simulink model "microcontroller"  (R2024b)
settings: Solver=FixedStepDiscrete  StartTime=0.0  StopTime=inf  RelTol=1e-3  EnableMultiTasking=on
values from neighbouring files (symbols this model uses):
  ac_curr_sens_offset = 1.252    [parameters.m]
  ac_curr_sens_slope = 20.39465588 * 1    (= 20.39465588)    [parameters.m]
  ac_volt_sens_offset = 1.51    [parameters.m]
  ac_volt_sens_slope = 33.33 * 1.00    (= 33.33)    [parameters.m]
  adc_intercept = 0.005546262    [parameters.m]
  adc_slope = 0.000812146    [parameters.m]
  adc_slope_volt = 0.00081 * 1.0    (= 0.00081)    [parameters.m]
  dc_volt_sens_offset = 0.981    [parameters.m]
  dc_volt_sens_slope = 15.122 * 1.0    (= 15.122)    [parameters.m]
  F28M35_freq = 150e6    (= 150000000)    [parameters.m]
  Fs = 20e3    (= 20000)    [parameters.m]
  KI_curr_d = KP_curr_d * Wp1_in    [pi_tuning.m]
  KI_curr_q = KI_curr_d    [pi_tuning.m]
  Ki_pll = 10000    [parameters.m]
  KI_q = C_q_ctrl.Ki    [pi_tuning.m]
  KI_volt = C_volt.Ki    [pi_tuning.m]
  KP_curr_d = Wbi / (DCGain_id * Wp1_in)    [pi_tuning.m]
  KP_curr_q = KP_curr_d    [pi_tuning.m]
  Kp_pll = 500    [parameters.m]
  KP_q = C_q_ctrl.Kp    [pi_tuning.m]
  KP_volt = C_volt.Kp    [pi_tuning.m]
  P = 0.041    [parameters.m]
  rdc = Vdc^2 / P    (= 21951.2195122)    [parameters.m]
  Vdc = 30    [parameters.m]
  wn = 2*pi*60    (= 376.991118431)    [parameters.m]
  Zl = w * Lc    (= 0.957557440814)    [parameters.m]
undefined symbols (not defined in the file or in its folder): Down, GPTRIP1SEL, TZ1, Up
libraries: slpidlib x4, c2802xlib x4, c2000lib x1
settings Model: ExtModeTrigDuration=8  Creator=Asus  LastModifiedBy=Asus
settings SolverCC: AutoInsertRateTranBlk=on
settings OptimizationCC: DefaultParameterBehavior=Inlined  DefaultUnderspecifiedDataType=single  EnhancedBackFolding=on  PassReuseOutputArgsAs=Individual arguments  MaxStackSize=768  OptimizeBlockOrder=speed  DifferentSizesBufferReuse=on  OptimizationCustomize=off  EfficientTunableParamExpr=on
settings DebuggingCC: ParameterTunabilityLossMsg=error
settings HardwareCC: ProdBitPerChar=16  ProdBitPerInt=16  ProdBitPerPointer=32  ProdBitPerSizeT=32  ProdBitPerPtrDiffT=32  ProdLargestAtomicInteger=Integer  ProdLargestAtomicFloat=None  ProdWordSize=16  ProdLongLongMode=on  ProdHWDeviceType=Texas Instruments->C2000
settings SFSimCC: MATLABDynamicMemAlloc=off
settings RTWCC: Description=Embedded Coder  SystemTargetFile=ert.tlc  HardwareBoard=TI Concerto F28M35x (C28x)  TemplateMakefile=ert_default_tmf  GenerateReport=on  Toolchain=Texas Instruments Code Composer Studio (C2000)  LaunchReport=on  CodeProfilingSaveOptions=MetricsOnly
settings RTWCC: CustomInitializer=|
  | InitAdc1();
  | EALLOW;
  | Adc1Regs.ADCCTL2.bit.ADCNONOVERLAP = 1; // Enable non-overlap mode i.e.
  | // conversion and future sampling
  | // events don’t overlap
  | Adc1Regs.ADCCTL1.bit.INTPULSEPOS = 1; // ADCINT1 trips after AdcResults latch
  | Adc1Regs.ADCSOC0CTL.bit.CHSEL = 0; // set SOC0 channel select to ADC1in_A0
  | AnalogSysctrlRegs.TRIG1SEL.all = 1; // Assigning TINT0 to ADC-TRIGGER 1
  | Adc1Regs.ADCSOC0CTL.bit.TRIGSEL = 5; // Set SOC0 start trigger to
  | // ADC Trigger 1 of the ADC
  | Adc1Regs.ADCSOC0CTL.bit.ACQPS = 6; // set SOC0 S/H Window to 7 ADC
  | // Clock Cycles, (6 ACQPS + 1)
  | EDIS;
  | 
  | EALLOW;
  | 
  | // SOC1: ADC1IN_A2
  | Adc1Regs.ADCSOC1CTL.bit.CHSEL = 2;        // Channel A2
  | Adc1Regs.ADCSOC1CTL.bit.TRIGSEL = 5;      // Trigger 1 (TINT0 from ePWM1)
  | Adc1Regs.ADCSOC1CTL.bit.ACQPS = 6;        // Acquisition window
  | 
  | // SOC2: ADC1IN_A3
  | Adc1Regs.ADCSOC2CTL.bit.CHSEL = 3;        // Channel A3
  | Adc1Regs.ADCSOC2CTL.bit.TRIGSEL = 5;      // Trigger 1 (TINT0 from ePWM1)
  | Adc1Regs.ADCSOC2CTL.bit.ACQPS = 6;        // Acquisition window
  | 
  | EDIS;
settings CodeAppCC: ForceParamTrailComments=on  IgnoreCustomStorageClasses=off  OperatorAnnotations=on  SimulinkDataObjDesc=on  SFDataObjDesc=on  InsertBlockDesc=on
settings ERTTargetCC: CodeReplacementLibrary=TI C28x  SupportContinuousTime=on  ExtModeTransport=4  ExtModeStaticAlloc=on  ExtModeAutomaticAllocSize=off  ExtModeStaticAllocSize=2000  ExtModeMexFile=ext_xcp  ExtModeIntrfLevel=Level2 - Open

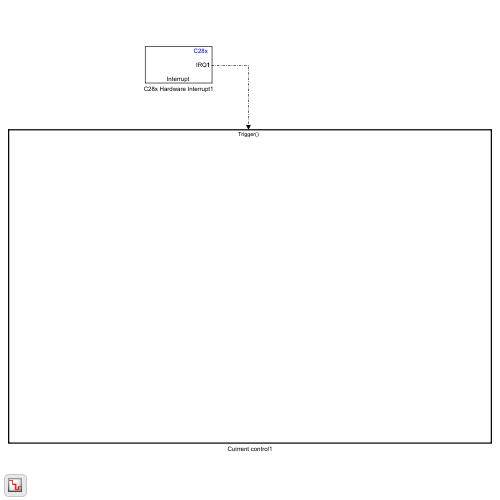
[thumbnail: Simulink's stored preview of the top-level diagram]
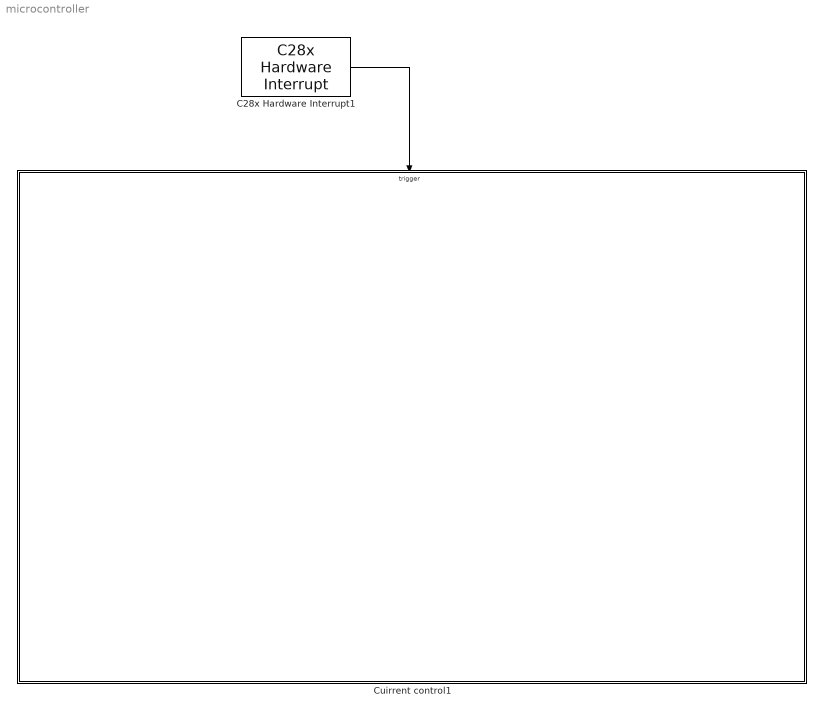
== system microcontroller ==
  C28x Hardware Interrupt1 : c2000lib/Scheduling/C28x Hardware Interrupt  irqnumbers=[1]  pienumbers=[1]  irqpriorities=[30]  irqpreempts=[0]  showinput=off  dspchiptype=C280X
  Cuirrent control1 : Subsystem  TreatAsAtomicUnit=on
  wires:
  C28x Hardware Interrupt1/1 -> Cuirrent control1/Trigger

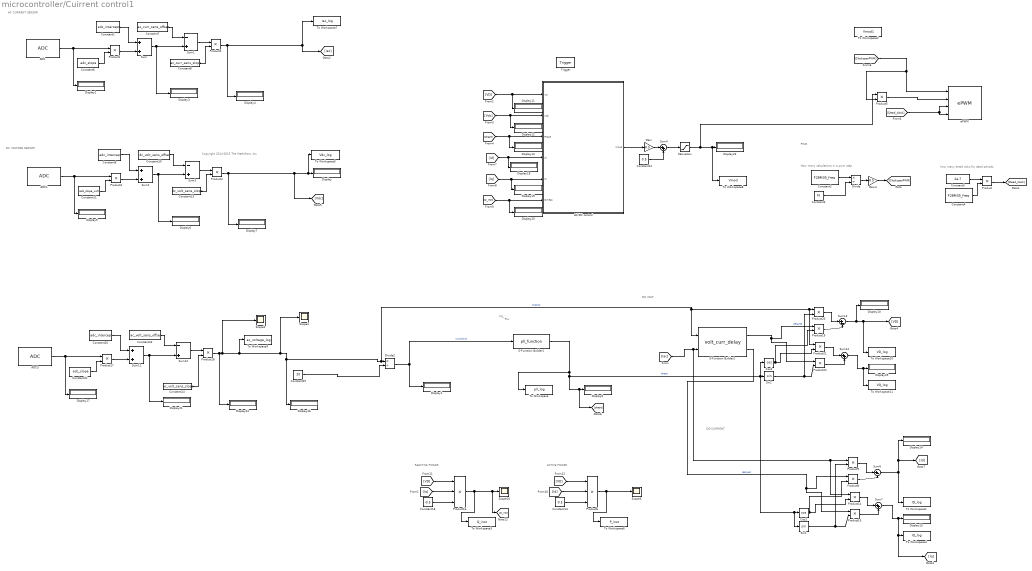
== system microcontroller/Cuirrent control1 ==
  note: PLL
  note: PLL
  note: how many break ticks for dead periods
  note: PWM
  note: How many calculations in a pwm step
  note: AC CURRENT SENSOR
  note: DC VOLTAGE SENSOR
  note: Copyright 2014-2015 The MathWors, Inc.
  note: DQ CURRENT
  note: REACTIVE POWER
  note: DQ VOLT
  note: ACTIVE POWER
  Trigger : TriggerPort  TriggerType=function-call  VariantControl=(inherit)  PortDimensions=1
  AC/DC control : Subsystem
  ADC : c2802xlib/ADC  blkParamProc=Concerto  ADCModule=1  samplingMode=Single sample mode  ADCResolution=12-bit (Single-ended input)  useSOC1=SOC0  useSOC2=SOC0_SOC1  SOCAcquisitionWindow=7  SOCTriggerSource=ePWM1_ADCSOCA  SOCInterruptTrigger=No ADCINT  Ts=-1  dType=uint16  postInterrupt=off  interruptSel=ADCINT1  ADCINTContinuous=off  endma=off  chdma=1  conv1=ADCINA0  conv2=ADCINA0 and ADCINB0  conv1_Type4=ADCIN0  conv2_Type4=ADCIN0 and ADCIN1
      settings: LibrarySourceBlock=f28M35x_C28x_lib/ADC
  ADC1 : c2802xlib/ADC  blkParamProc=Concerto  ADCModule=1  samplingMode=Single sample mode  ADCResolution=12-bit (Single-ended input)  useSOC1=SOC1  useSOC2=SOC0_SOC1  SOCAcquisitionWindow=7  SOCTriggerSource=ePWM1_ADCSOCA  SOCInterruptTrigger=No ADCINT  Ts=-1  dType=uint16  postInterrupt=off  interruptSel=ADCINT1  ADCINTContinuous=off  endma=off  chdma=1  conv1=ADCINA2  conv2=ADCINA0 and ADCINB0  conv1_Type4=ADCIN0  conv2_Type4=ADCIN0 and ADCIN1
      settings: LibrarySourceBlock=f28M35x_C28x_lib/ADC
  ADC3 : c2802xlib/ADC  blkParamProc=Concerto  ADCModule=1  samplingMode=Single sample mode  ADCResolution=12-bit (Single-ended input)  useSOC1=SOC2  useSOC2=SOC0_SOC1  SOCAcquisitionWindow=7  SOCTriggerSource=ePWM1_ADCSOCA  SOCInterruptTrigger=No ADCINT  Ts=-1  dType=uint16  postInterrupt=on  interruptSel=ADCINT1  ADCINTContinuous=off  endma=off  chdma=1  conv1=ADCINA3  conv2=ADCINA0 and ADCINB0  conv1_Type4=ADCIN0  conv2_Type4=ADCIN0 and ADCIN1
      settings: LibrarySourceBlock=f28M35x_C28x_lib/ADC
  Constant1 : Constant  Value=adc_intercept
  Constant10 : Constant  Value=dc_volt_sens_offset
  Constant11 : Constant  Value=adc_slope_volt
  Constant12 : Constant  Value=0.5
  Constant13 : Constant  Value=dc_volt_sens_slope
  Constant14 : Constant  Value=0.5
  Constant18 : Constant  Value=-0.5
  Constant2 : Constant  Value=F28M35_freq
  Constant20 : Constant  Value=adc_intercept
  Constant21 : Constant  Value=adc_slope
  Constant23 : Constant  Value=ac_volt_sens_offset
  Constant24 : Constant  Value=ac_volt_sens_slope
  Constant25 : Constant  Value=20
  Constant3 : Constant  Value=Fs
  Constant4 : Constant  Value=F28M35_freq
  Constant5 : Constant  Value=2e-7
  Constant6 : Constant  Value=adc_slope
  Constant7 : Constant  Value=ac_curr_sens_offset
  Constant8 : Constant  Value=ac_curr_sens_slope
  Constant9 : Constant  Value=adc_intercept
  Cos1 : Trigonometry  Operator=cos
  Cos2 : Trigonometry  Operator=cos
  Display{,1..8,10..23,25} (24 alike) : Display
  Divide : Product  Inputs=*/
  Divide2 : Product  Inputs=*/
  Gain : Gain  Gain=0.5
  Gain4 : Gain  Gain=0.5
  Product{,1..5,8..9,14..15,17..22} (16 alike) : Product
  Product16 : Product  Inputs=3
  Product6 : Product  Inputs=3
  S-Function Builder1 : S-Function  FunctionName=pll_function  Parameters=Kp_pll,Ki_pll,wn  SFunctionModules=pll_function_wrapper.c  SFunctionDeploymentMode=off  EnableBusSupport=off  mask(S-Function Builder){}
      mask help: Simulink:masks:SFunctionBuilder_MD
      mask init:
      | val = [[.9  0.75 0.75 1 1 .9 .9 1]',[1 1 0.75 0.75 .9 .9 1 .9]'];try , sys = get_param(gcb,'SfunBuilderFcnName');if isempty(sys), sys = get_param(gcb,'FunctionName'); end,catch, sys = get_param(gcb,'FunctionName'); end
      settings: CopyFcn=set_param(gcbh,'LinkStatus','none')  OpenFcn=sfunctionwizard(gcbh)
      mask Display:
      | plot(val(:,1),val(:,2))
      | disp(sys)
      | port_label('input',1,sprintf('%s', 'Vac'),'interpreter','tex')
      | port_label('output',1,sprintf('%s', 'phase'),'interpreter','tex')
  S-Function Builder2 : S-Function  FunctionName=volt_curr_delay  SFunctionModules=volt_curr_delay_wrapper.c  SFunctionDeploymentMode=off  EnableBusSupport=off  mask(S-Function Builder){}
      mask help: Simulink:masks:SFunctionBuilder_MD
      mask init: same as microcontroller/Cuirrent control1/S-Function Builder1
      settings: CopyFcn=set_param(gcbh,'LinkStatus','none')  OpenFcn=sfunctionwizard(gcbh)
      mask Display:
      | plot(val(:,1),val(:,2))
      | disp(sys)
      | port_label('input',1,sprintf('%s', 'Vorigin'),'interpreter','tex')
      | port_label('input',2,sprintf('%s', 'Iorigin'),'interpreter','tex')
      | port_label('output',1,sprintf('%s', 'Vdelay'),'interpreter','tex')
      | port_label('output',2,sprintf('%s', 'Idelay'),'interpreter','tex')
  Saturation : Saturate  UpperLimit=1  LowerLimit=0
  Scope{1..3,10} (4 alike) : Scope
  Sin1 : Trigonometry
  Sin2 : Trigonometry
  Sum : Sum
  Sum1 : Sum  Inputs=-+
  Sum11 : Sum
  Sum12 : Sum  Inputs=-+
  Sum13 : Sum  Inputs=|+-
  Sum14 : Sum  Inputs=|++
  Sum2 : Sum
  Sum3 : Sum  Inputs=-+
  Sum4 : Sum  Inputs=|++
  Sum6 : Sum  Inputs=|+-
  Sum7 : Sum  Inputs=|++
  To Workspace : ToWorkspace  VariableName=pll_log  SampleTime=-1
      settings: MaxDataPoints=5000
  To Workspace1 : ToWorkspace  VariableName=ID_log  SampleTime=-1
      settings: MaxDataPoints=5000
  To Workspace10 : ToWorkspace  VariableName=VD_log  SampleTime=-1
      settings: MaxDataPoints=5000
  To Workspace11 : ToWorkspace  VariableName=VQ_log  SampleTime=-1
      settings: MaxDataPoints=5000
  To Workspace2 : ToWorkspace  VariableName=Vmod1  SampleTime=-1
      settings: MaxDataPoints=5000
  To Workspace3 : ToWorkspace  VariableName=Q_inst  SampleTime=-1
      settings: MaxDataPoints=5000
  To Workspace4 : ToWorkspace  VariableName=IQ_log  SampleTime=-1
      settings: MaxDataPoints=5000
  To Workspace5 : ToWorkspace  VariableName=Vdc_log  SampleTime=-1
      settings: MaxDataPoints=5000
  To Workspace6 : ToWorkspace  VariableName=P_inst  SampleTime=-1
      settings: MaxDataPoints=5000
  To Workspace7 : ToWorkspace  VariableName=Iac_log  SampleTime=-1
      settings: MaxDataPoints=5000
  To Workspace8 : ToWorkspace  VariableName=Vmod  SampleTime=-1
      settings: MaxDataPoints=5000
  To Workspace9 : ToWorkspace  VariableName=ac_voltage_log  SampleTime=-1
      settings: MaxDataPoints=5000
  ePWM : c2802xlib/ePWM  PwmType=Concerto  useModule=ePWM1  ePWMxLINKTBPRD=Not Linked  periodUnits=Clock cycles  timerSource=Input port  timerPeriod_clk=3750  timerPeriod_sec=5e-5  tbshadow=Counter equals to zero  countingMode=Up-Down  phaseActiveEnable=Disable  phaseDirection=Count down after sync  phaseActive=0  synchronizationEnable=off  dcaevt1Sync=off  dcbevt1Sync=off  synchronizationOption=Disable  dcbevt1SyncOut=off  dcaevt1SyncOut=off  cmpdSyncOut=off  cmpcSyncOut=off  cmpbSyncOut=off  zeroSyncOut=off  swfSyncOut=off  perSynchronizationOption=Counter equals to period (CTR=PRD)  clockPrescale=1  HSclockPrescale=1  enswap=off  ePWMxAStatus=on  ePWMxAactionLogic1=Do nothing  ePWMxAactionLogic2=Do nothing  ePWMxAactionLogic3=Clear  ePWMxAactionLogic4=Set  ePWMxAactionLogic5=Do nothing  ePWMxAactionLogic6=Do nothing  ePWMxACSFenable=off  ePWMxACSFvalue=Forcing disable  ePWMxASFreload=Zero  ePWMxBStatus=on  ePWMxBactionLogic1=Do nothing  ePWMxBactionLogic2=Do nothing  ePWMxBactionLogic3=Set  ePWMxBactionLogic4=Clear  ePWMxBactionLogic5=Clear  ePWMxBactionLogic6=Set  ePWMxBCSFenable=off  ePWMxBCSFvalue=Forcing disable  ePWMxBSFreload=Zero  ePWNxBOutWay=on  ePWMxLINKCMPA=Not Linked  CMPAUnits=Clock cycles  CMPASource=Input port  CMPAValue_per=50  CMPAValue_clk=0  enCMPAshadow=Counter equals to zero (CTR=Zero)  ePWMxLINKCMPB=Not Linked  CMPBUnits=Clock cycles  CMPBSource=Specify via dialog  CMPBValue_per=50  CMPBValue_clk=0  enCMPBshadow=Counter equals to zero (CTR=Zero)  ePWMxLINKCMPC=Not Linked  CMPCUnits=Clock cycles  CMPCSource=Specify via dialog  CMPCValue_per=50  CMPCValue_clk=0  enCMPCshadow=Counter equals to zero (CTR=Zero)  ePWMxLINKCMPD=Not Linked  CMPDUnits=Clock cycles  CMPDSource=Specify via dialog  CMPDValue_per=50  CMPDValue_clk=32000  enCMPDshadow=Counter equals to zero (CTR=Zero)  enableDBePWMxA=on  enableDBePWMxB=on  enhalfcycle=off  DBpolarity=Active high complementary (AHC)  DBedgeDelay=Positive  DBSource_ePWMxA=ePWMxA  DBSource_ePWMxB=ePWMxA  DBPeriodUnits=Clock cycles  DBperiodSource=Input port  REDperiod=220  FEDperiod=220  REDperiod_sec=0  FEDperiod_sec=0  LoadModeDBRED=Immediate without using shadow  LoadModeDBFED=Immediate without using shadow  adcstartModuleA=on  adcrequestEventA=First event  adcstartEventA=Digital Compare Module A Event 1 start of conversion (DCAEVT1.soc)  adcstartEventA_type2=Counter equals to period (CTR=PRD)  adcstartModuleB=off  adcrequestEventB=First event  adcstartEventB=Counter equals to zero (CTR=Zero)  adcstartEventB_type2=Counter equals to zero (CTR=Zero)  intEn=off  intPrd=First event  intSel=Counter equals to zero (CTR=Zero)  intSel_type2=Counter equals to zero (CTR=Zero)  hrpe=off  enHRPWM=off  HRPWM_LoadMode=Counter equals to period (CTR=PRD)  HRPWM_CTLMode=Duty or Period control mode  HRPWM_EDGMode=Both edge  hrpeb=off  enHRPWMB=off  HRPWM_LoadModeB=Counter equals to zero (CTR=ZERO)  HRPWM_CTLModeB=Duty or Period control mode  HRPWM_EDGModeB=Both edge  enHRDBRED=off  enHRDBFED=off  enSFO=on  enautoconv=on  chopperEnable=off  chopperFrequency=1  chopperFirstwidth=1  chopperDuty=12.5%  tripZonesource=Specify via dialog  tzselOSHT1=off  tzselOSHT2=off  tzselOSHT3=off  tzselOSHT4=off  tzselOSHT5=off  tzselOSHT6=off  tzselOSHDCAEV1=off  tzselOSHDCBEV1=off  tzselCBC1=off  tzselCBC2=off  tzselCBC3=off  tzselCBC4=off  tzselCBC5=off  tzselCBC6=off  tzselCBCDCAEV2=off  tzselCBCDCBEV2=off  enTzOstIntr=off  enTzCbcIntr=off  enTzDCAEVT1Intr=off  enTzDCAEVT2Intr=off  enTzDCBEVT1Intr=off  enTzDCBEVT2Intr=off  tzclrCBCLatch=Counter equals to zero (CTR=Zero)  ePWMxAforced=Low  ePWMxBforced=Low  DCAEVT1forced=No action  DCBEVT1forced=No action  DCAEVT2forced=No action  DCBEVT2forced=No action  dcah=Trip Zone 1 input (TZ1)  dcal=Trip Zone 2 input (TZ2)  dcbh=Trip Zone 1 input (TZ1)  dcbl=Trip Zone 2 input (TZ2)  dcah_type2=GPTRIP1SEL/(TZ1)  dcal_type2=GPTRIP1SEL/(TZ1)  dcbh_type2=GPTRIP1SEL/(TZ1)  dcbl_type2=GPTRIP1SEL/(TZ1)  gendcaevt1=Event disabled  gendcaevt2=Event disabled  gendcbevt1=Event disabled  gendcbevt2=Event disabled  dcaevt1src=DCAEVT1 with sync  dcaevt2src=DCAEVT2 with sync  dcbevt1src=DCBEVT1 with sync  dcbevt2src=DCBEVT2 with sync  pulsesel=Counter equals to zero (CTR=Zero)  blankinv=off  blankoffset=0  blankwidth=0  evsrcsel=Filtered version of DCAEVT1 (DCAEVT1FILT)  encape=off
      settings: LibrarySourceBlock=f28M35x_C28x_lib/ePWM
  wires:
  Constant4/1 -> Product/2
  Divide/1 -> Gain4/1
  Gain4/1 -> [ClocksperPWM]
  Constant5/1 -> Product/1
  Constant2/1 -> Divide/1
  Constant3/1 -> Divide/2
  Product/1 -> [Dead_clock]
  [Dead_clock] -> ePWM/3, ePWM/4
  Product5/1 -> ePWM/2
  [ClocksperPWM] -> Product5/2, ePWM/1
  ADC/1 -> Product1/1, Display2/1
  Constant8/1 -> Product2/2
  Sum/1 -> Sum1/2, Display3/1
  Constant6/1 -> Product1/2
  Sum1/1 -> Product2/1
  Product1/1 -> Sum/2
  Constant7/1 -> Sum1/1
  Product2/1 -> [Iac], To Workspace7/1, Display4/1
  Constant1/1 -> Sum/1
  Sum2/1 -> Sum3/2, Display6/1
  Constant13/1 -> Product4/2
  Constant10/1 -> Sum3/1
  ADC1/1 -> Product3/1, Display5/1
  Product3/1 -> Sum2/2
  Constant11/1 -> Product3/2
  Sum3/1 -> Product4/1
  Product4/1 -> [Vdc], To Workspace5/1, Display/1, Display7/1
  Constant9/1 -> Sum2/1
  Constant20/1 -> Sum11/1
  Product17/1 -> Sum11/2
  ADC3/1 -> Product17/1, Display17/1
  Constant21/1 -> Product17/2
  Constant25/1 -> Divide2/2
  Product18/1 -> Display22/1, To Workspace9/1, Scope1/1, Product21/1, Product20/1, S-Function Builder2/1, Divide2/1, Display16/1, Scope2/1  "original"
  Sum12/1 -> Product18/1
  Divide2/1 -> S-Function Builder1/1, Display1/1  "Vd control"
  Sum11/1 -> Sum12/2, Display21/1
  Constant23/1 -> Sum12/1
  Constant24/1 -> Product18/2
  S-Function Builder1/1 -> Cos2/1, Sin2/1, Sin1/1, Cos1/1, [phase], Display8/1, To Workspace/1  "phase"
  Product21/1 -> Sum14/1
  Cos1/1 -> Product8/2, Product14/2
  Product8/1 -> Sum6/2
  Sum14/1 -> To Workspace11/1, Display25/1
  Sum6/1 -> [Id], Display14/1, To Workspace1/1
  Sin2/1 -> Product20/2, Product22/2
  Product19/1 -> Sum13/2
  Product14/1 -> Sum7/1
  Sum13/1 -> Display10/1, [VD], To Workspace10/1
  Product20/1 -> Sum13/1
  Product9/1 -> Sum6/1
  Product22/1 -> Sum14/2
  Cos2/1 -> Product19/2, Product21/2
  Product15/1 -> Sum7/2
  S-Function Builder2/1 -> Product22/1, Product19/1  "delayed"
  Sin1/1 -> Product15/2, Product9/2
  S-Function Builder2/2 -> Product15/1, Product8/1  "delayed"
  Sum7/1 -> [Iq], To Workspace4/1, Display15/1
  [Iac] -> Product14/1, Product9/1, S-Function Builder2/2
  [VD] -> Product16/1
  [Iq] -> Product16/2
  Constant18/1 -> Product16/3
  Product16/1 -> To Workspace3/1, [Q_inst], Scope10/1
  [Id] -> Display18/1, AC/DC control/4(Id)
  AC/DC control/1(Vmod) -> Gain/1
  [Iq] -> Display19/1, AC/DC control/5(Iq)
  [VD] -> Display11/1, AC/DC control/1(Vd)
  Constant12/1 -> Sum4/2
  Gain/1 -> Sum4/1
  [Q_inst] -> Display20/1, AC/DC control/6(Qmeas)
  Sum4/1 -> Saturation/1
  [Vdc] -> Display12/1, AC/DC control/2(Vdc)
  [phase] -> Display13/1, AC/DC control/3(Phase)
  Product6/1 -> To Workspace6/1, Scope3/1
  Constant14/1 -> Product6/3
  [Id] -> Product6/2
  [VD] -> Product6/1
  Saturation/1 -> Product5/1, To Workspace8/1, Display23/1

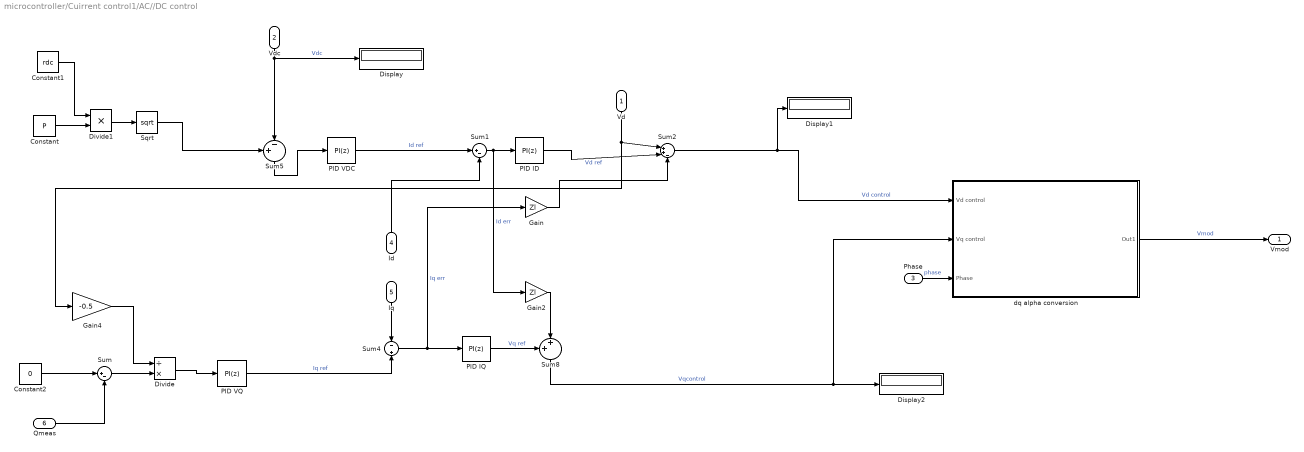
== system microcontroller/Cuirrent control1/AC//DC control ==
  Vd : Inport
  Vdc : Inport  Port=2
  Phase : Inport  Port=3
  Id : Inport  Port=4
  Iq : Inport  Port=5
  Qmeas : Inport  Port=6
  Constant : Constant  Value=P
  Constant1 : Constant  Value=rdc
  Constant2 : Constant  Value=0
  Display : Display
  Display1 : Display
  Display2 : Display
  Divide : Product  Inputs=/*
  Divide1 : Product  Inputs=**
  Gain : Gain  Gain=Zl
  Gain2 : Gain  Gain=Zl
  Gain4 : Gain  Gain=-0.5
  "PID ID " : slpidlib/PID Controller  Controller=PI  Form=Parallel  TimeDomain=Discrete-time  UseExternalTs=off  SampleTime=-1  IntegratorMethod=Forward Euler  FilterMethod=Forward Euler  ControllerParametersSource=internal  P=KP_curr_d  I=KI_curr_d  UseKiTs=off  D=0  UseExternalDerivativeSource=off  N=100  UseFilter=on  TunerSelectOption=Transfer Function Based (PID Tuner App)  InitialConditionSource=internal  InitialConditionForIntegrator=0  InitialConditionForFilter=0  DifferentiatorICPrevScaledInput=0  ExternalReset=none  TrackingMode=off  Kt=1  LimitOutput=off  SatLimitsSource=internal  UpperSaturationLimit=200  LowerSaturationLimit=-inf  LinearizeAsGain=on  AntiWindupMode=none  Kb=1  LimitIntegrator=off  UpperIntegratorSaturationLimit=inf  LowerIntegratorSaturationLimit=-inf  POutMin=[]  POutMax=[]  IOutMin=[]  IOutMax=[]  DOutMin=[]  DOutMax=[]  NOutMin=[]  NOutMax=[]  SumOutMin=[]  SumOutMax=[]  SaturationOutMin=[]  SaturationOutMax=[]  PParamMin=[]  PParamMax=[]  IParamMin=[]  IParamMax=[]  DParamMin=[]  DParamMax=[]  NParamMin=[]  NParamMax=[]  KbParamMin=[]  KbParamMax=[]  KtParamMin=[]  KtParamMax=[]  KbOutMin=[]  KbOutMax=[]  KtOutMin=[]  KtOutMax=[]  IntegratorOutMin=[]  IntegratorOutMax=[]  FilterOutMin=[]  FilterOutMax=[]  SumI1OutMin=[]  SumI1OutMax=[]  SumI2OutMin=[]  SumI2OutMax=[]  SumI3OutMin=[]  SumI3OutMax=[]  SumI4OutMin=[]  SumI4OutMax=[]  SumDOutMin=[]  SumDOutMax=[]  DifferentiatorOutMin=[]  DifferentiatorOutMax=[]  FilterDiffOutCoefMin=[]  FilterDiffOutCoefMax=[]  ReciprocalOutMin=[]  ReciprocalOutMax=[]  SumDenOutMin=[]  SumDenOutMax=[]  SumNumOutMin=[]  SumNumOutMax=[]  DivideOutMin=[]  DivideOutMax=[]  UdiffTsProdOutMin=[]  UdiffTsProdOutMax=[]  NTsProdOutMin=[]  NTsProdOutMax=[]  UintegralTsProdOutMin=[]  UintegralTsProdOutMax=[]  UngainTsProdOutMin=[]  UngainTsProdOutMax=[]  ClampingZeroOutDataTypeStr=Inherit: Inherit via back propagation  ClampingZeroOutMin=[]  ClampingZeroOutMax=[]  FilterDenConstantOutDataTypeStr=Inherit: Inherit via back propagation  FilterDenConstantOutMin=[]  FilterDenConstantOutMax=[]  PCopyOutDataTypeStr=Inherit: Inherit via back propagation  PCopyOutMin=[]  PCopyOutMax=[]  NCopyOutDataTypeStr=Inherit: Inherit via back propagation  NCopyOutMin=[]  NCopyOutMax=[]  IntegratorContinuousStateAttributes=''  IntegratorStateMustResolveToSignalObject=off  IntegratorRTWStateStorageClass=Auto  FilterContinuousStateAttributes=''  FilterStateMustResolveToSignalObject=off  FilterRTWStateStorageClass=Auto  ParallelPVariant=InternalParameters  IdealPVariant=Disabled  IVariant=InternalParameters  DVariant=Disabled  IntegratorVariant=Discrete  SatVariant=Disabled  AWVariant=Passthrough  PCopyVariant=Disabled  TRVariant=Disabled  FdbkBlocksVariant=Forward  IdealPFdbkVariant=Disabled  SatFdbkVariant=Disabled  DerivativeFilterVariant=Disabled  NVariant=Disabled  NCopyVariant=Disabled_SignalSpec  FilterICVariant=Disabled  IntegratorICVariant=InternalICs  ExternalResetVariant=Disabled  TRSumVariant=Passthrough  SumFdbkVariant=Disabled  SumVariant=Sum_PI  TsampFilterVariant=InternalTs  TsampNgainVariant=Passthrough  TsampIntegralVariant=Disabled_SignalSpec  ExternalSaturationOutDataTypeStr=Inherit: Same as second input  DerivativeSourceVariant=Disabled  PreIntVariant=InternalPreInt
  PID IQ : slpidlib/PID Controller  Controller=PI  Form=Parallel  TimeDomain=Discrete-time  UseExternalTs=off  SampleTime=-1  IntegratorMethod=Forward Euler  FilterMethod=Forward Euler  ControllerParametersSource=internal  P=KP_curr_q  I=KI_curr_q  UseKiTs=off  D=0  UseExternalDerivativeSource=off  N=100  UseFilter=on  TunerSelectOption=Transfer Function Based (PID Tuner App)  InitialConditionSource=internal  InitialConditionForIntegrator=0  InitialConditionForFilter=0  DifferentiatorICPrevScaledInput=0  ExternalReset=none  TrackingMode=off  Kt=1  LimitOutput=off  SatLimitsSource=internal  UpperSaturationLimit=15  LowerSaturationLimit=-15  LinearizeAsGain=on  AntiWindupMode=none  Kb=1  LimitIntegrator=off  UpperIntegratorSaturationLimit=inf  LowerIntegratorSaturationLimit=-inf  POutMin=[]  POutMax=[]  IOutMin=[]  IOutMax=[]  DOutMin=[]  DOutMax=[]  NOutMin=[]  NOutMax=[]  SumOutMin=[]  SumOutMax=[]  SaturationOutMin=[]  SaturationOutMax=[]  PParamMin=[]  PParamMax=[]  IParamMin=[]  IParamMax=[]  DParamMin=[]  DParamMax=[]  NParamMin=[]  NParamMax=[]  KbParamMin=[]  KbParamMax=[]  KtParamMin=[]  KtParamMax=[]  KbOutMin=[]  KbOutMax=[]  KtOutMin=[]  KtOutMax=[]  IntegratorOutMin=[]  IntegratorOutMax=[]  FilterOutMin=[]  FilterOutMax=[]  SumI1OutMin=[]  SumI1OutMax=[]  SumI2OutMin=[]  SumI2OutMax=[]  SumI3OutMin=[]  SumI3OutMax=[]  SumI4OutMin=[]  SumI4OutMax=[]  SumDOutMin=[]  SumDOutMax=[]  DifferentiatorOutMin=[]  DifferentiatorOutMax=[]  FilterDiffOutCoefMin=[]  FilterDiffOutCoefMax=[]  ReciprocalOutMin=[]  ReciprocalOutMax=[]  SumDenOutMin=[]  SumDenOutMax=[]  SumNumOutMin=[]  SumNumOutMax=[]  DivideOutMin=[]  DivideOutMax=[]  UdiffTsProdOutMin=[]  UdiffTsProdOutMax=[]  NTsProdOutMin=[]  NTsProdOutMax=[]  UintegralTsProdOutMin=[]  UintegralTsProdOutMax=[]  UngainTsProdOutMin=[]  UngainTsProdOutMax=[]  ClampingZeroOutDataTypeStr=Inherit: Inherit via back propagation  ClampingZeroOutMin=[]  ClampingZeroOutMax=[]  FilterDenConstantOutDataTypeStr=Inherit: Inherit via back propagation  FilterDenConstantOutMin=[]  FilterDenConstantOutMax=[]  PCopyOutDataTypeStr=Inherit: Inherit via back propagation  PCopyOutMin=[]  PCopyOutMax=[]  NCopyOutDataTypeStr=Inherit: Inherit via back propagation  NCopyOutMin=[]  NCopyOutMax=[]  IntegratorContinuousStateAttributes=''  IntegratorStateMustResolveToSignalObject=off  IntegratorRTWStateStorageClass=Auto  FilterContinuousStateAttributes=''  FilterStateMustResolveToSignalObject=off  FilterRTWStateStorageClass=Auto  ParallelPVariant=InternalParameters  IdealPVariant=Disabled  IVariant=InternalParameters  DVariant=Disabled  IntegratorVariant=Discrete  SatVariant=Disabled  AWVariant=Passthrough  PCopyVariant=Disabled  TRVariant=Disabled  FdbkBlocksVariant=Forward  IdealPFdbkVariant=Disabled  SatFdbkVariant=Disabled  DerivativeFilterVariant=Disabled  NVariant=Disabled  NCopyVariant=Disabled_SignalSpec  FilterICVariant=Disabled  IntegratorICVariant=InternalICs  ExternalResetVariant=Disabled  TRSumVariant=Passthrough  SumFdbkVariant=Disabled  SumVariant=Sum_PI  TsampFilterVariant=InternalTs  TsampNgainVariant=Passthrough  TsampIntegralVariant=Disabled_SignalSpec  ExternalSaturationOutDataTypeStr=Inherit: Same as second input  DerivativeSourceVariant=Disabled  PreIntVariant=InternalPreInt
  PID VDC : slpidlib/PID Controller  Controller=PI  Form=Parallel  TimeDomain=Discrete-time  UseExternalTs=off  SampleTime=-1  IntegratorMethod=Forward Euler  FilterMethod=Forward Euler  ControllerParametersSource=internal  P=-KP_volt  I=-KI_volt  UseKiTs=off  D=0  UseExternalDerivativeSource=off  N=100  UseFilter=on  TunerSelectOption=Frequency Response Based  InitialConditionSource=internal  InitialConditionForIntegrator=0  InitialConditionForFilter=0  DifferentiatorICPrevScaledInput=0  ExternalReset=none  TrackingMode=off  Kt=1  LimitOutput=off  SatLimitsSource=internal  UpperSaturationLimit=16  LowerSaturationLimit=-16  LinearizeAsGain=on  AntiWindupMode=none  Kb=1  LimitIntegrator=off  UpperIntegratorSaturationLimit=inf  LowerIntegratorSaturationLimit=-inf  POutMin=[]  POutMax=[]  IOutMin=[]  IOutMax=[]  DOutMin=[]  DOutMax=[]  NOutMin=[]  NOutMax=[]  SumOutMin=[]  SumOutMax=[]  SaturationOutMin=[]  SaturationOutMax=[]  PParamMin=[]  PParamMax=[]  IParamMin=[]  IParamMax=[]  DParamMin=[]  DParamMax=[]  NParamMin=[]  NParamMax=[]  KbParamMin=[]  KbParamMax=[]  KtParamMin=[]  KtParamMax=[]  KbOutMin=[]  KbOutMax=[]  KtOutMin=[]  KtOutMax=[]  IntegratorOutMin=[]  IntegratorOutMax=[]  FilterOutMin=[]  FilterOutMax=[]  SumI1OutMin=[]  SumI1OutMax=[]  SumI2OutMin=[]  SumI2OutMax=[]  SumI3OutMin=[]  SumI3OutMax=[]  SumI4OutMin=[]  SumI4OutMax=[]  SumDOutMin=[]  SumDOutMax=[]  DifferentiatorOutMin=[]  DifferentiatorOutMax=[]  FilterDiffOutCoefMin=[]  FilterDiffOutCoefMax=[]  ReciprocalOutMin=[]  ReciprocalOutMax=[]  SumDenOutMin=[]  SumDenOutMax=[]  SumNumOutMin=[]  SumNumOutMax=[]  DivideOutMin=[]  DivideOutMax=[]  UdiffTsProdOutMin=[]  UdiffTsProdOutMax=[]  NTsProdOutMin=[]  NTsProdOutMax=[]  UintegralTsProdOutMin=[]  UintegralTsProdOutMax=[]  UngainTsProdOutMin=[]  UngainTsProdOutMax=[]  ClampingZeroOutDataTypeStr=Inherit: Inherit via back propagation  ClampingZeroOutMin=[]  ClampingZeroOutMax=[]  FilterDenConstantOutDataTypeStr=Inherit: Inherit via back propagation  FilterDenConstantOutMin=[]  FilterDenConstantOutMax=[]  PCopyOutDataTypeStr=Inherit: Inherit via back propagation  PCopyOutMin=[]  PCopyOutMax=[]  NCopyOutDataTypeStr=Inherit: Inherit via back propagation  NCopyOutMin=[]  NCopyOutMax=[]  IntegratorContinuousStateAttributes=''  IntegratorStateMustResolveToSignalObject=off  IntegratorRTWStateStorageClass=Auto  FilterContinuousStateAttributes=''  FilterStateMustResolveToSignalObject=off  FilterRTWStateStorageClass=Auto  ParallelPVariant=InternalParameters  IdealPVariant=Disabled  IVariant=InternalParameters  DVariant=Disabled  IntegratorVariant=Discrete  SatVariant=Disabled  AWVariant=Passthrough  PCopyVariant=Disabled  TRVariant=Disabled  FdbkBlocksVariant=Forward  IdealPFdbkVariant=Disabled  SatFdbkVariant=Disabled  DerivativeFilterVariant=Disabled  NVariant=Disabled  NCopyVariant=Disabled_SignalSpec  FilterICVariant=Disabled  IntegratorICVariant=InternalICs  ExternalResetVariant=Disabled  TRSumVariant=Passthrough  SumFdbkVariant=Disabled  SumVariant=Sum_PI  TsampFilterVariant=InternalTs  TsampNgainVariant=Passthrough  TsampIntegralVariant=Disabled_SignalSpec  ExternalSaturationOutDataTypeStr=Inherit: Same as second input  DerivativeSourceVariant=Disabled  PreIntVariant=InternalPreInt
  PID VQ : slpidlib/PID Controller  Controller=PI  Form=Parallel  TimeDomain=Discrete-time  UseExternalTs=off  SampleTime=-1  IntegratorMethod=Forward Euler  FilterMethod=Forward Euler  ControllerParametersSource=internal  P=KP_q+0.08  I=KI_q  UseKiTs=off  D=0  UseExternalDerivativeSource=off  N=100  UseFilter=on  TunerSelectOption=Frequency Response Based  InitialConditionSource=internal  InitialConditionForIntegrator=0  InitialConditionForFilter=0  DifferentiatorICPrevScaledInput=0  ExternalReset=none  TrackingMode=off  Kt=1  LimitOutput=off  SatLimitsSource=internal  UpperSaturationLimit=16  LowerSaturationLimit=-16  LinearizeAsGain=on  AntiWindupMode=none  Kb=1  LimitIntegrator=off  UpperIntegratorSaturationLimit=inf  LowerIntegratorSaturationLimit=-inf  POutMin=[]  POutMax=[]  IOutMin=[]  IOutMax=[]  DOutMin=[]  DOutMax=[]  NOutMin=[]  NOutMax=[]  SumOutMin=[]  SumOutMax=[]  SaturationOutMin=[]  SaturationOutMax=[]  PParamMin=[]  PParamMax=[]  IParamMin=[]  IParamMax=[]  DParamMin=[]  DParamMax=[]  NParamMin=[]  NParamMax=[]  KbParamMin=[]  KbParamMax=[]  KtParamMin=[]  KtParamMax=[]  KbOutMin=[]  KbOutMax=[]  KtOutMin=[]  KtOutMax=[]  IntegratorOutMin=[]  IntegratorOutMax=[]  FilterOutMin=[]  FilterOutMax=[]  SumI1OutMin=[]  SumI1OutMax=[]  SumI2OutMin=[]  SumI2OutMax=[]  SumI3OutMin=[]  SumI3OutMax=[]  SumI4OutMin=[]  SumI4OutMax=[]  SumDOutMin=[]  SumDOutMax=[]  DifferentiatorOutMin=[]  DifferentiatorOutMax=[]  FilterDiffOutCoefMin=[]  FilterDiffOutCoefMax=[]  ReciprocalOutMin=[]  ReciprocalOutMax=[]  SumDenOutMin=[]  SumDenOutMax=[]  SumNumOutMin=[]  SumNumOutMax=[]  DivideOutMin=[]  DivideOutMax=[]  UdiffTsProdOutMin=[]  UdiffTsProdOutMax=[]  NTsProdOutMin=[]  NTsProdOutMax=[]  UintegralTsProdOutMin=[]  UintegralTsProdOutMax=[]  UngainTsProdOutMin=[]  UngainTsProdOutMax=[]  ClampingZeroOutDataTypeStr=Inherit: Inherit via back propagation  ClampingZeroOutMin=[]  ClampingZeroOutMax=[]  FilterDenConstantOutDataTypeStr=Inherit: Inherit via back propagation  FilterDenConstantOutMin=[]  FilterDenConstantOutMax=[]  PCopyOutDataTypeStr=Inherit: Inherit via back propagation  PCopyOutMin=[]  PCopyOutMax=[]  NCopyOutDataTypeStr=Inherit: Inherit via back propagation  NCopyOutMin=[]  NCopyOutMax=[]  IntegratorContinuousStateAttributes=''  IntegratorStateMustResolveToSignalObject=off  IntegratorRTWStateStorageClass=Auto  FilterContinuousStateAttributes=''  FilterStateMustResolveToSignalObject=off  FilterRTWStateStorageClass=Auto  ParallelPVariant=InternalParameters  IdealPVariant=Disabled  IVariant=InternalParameters  DVariant=Disabled  IntegratorVariant=Discrete  SatVariant=Disabled  AWVariant=Passthrough  PCopyVariant=Disabled  TRVariant=Disabled  FdbkBlocksVariant=Forward  IdealPFdbkVariant=Disabled  SatFdbkVariant=Disabled  DerivativeFilterVariant=Disabled  NVariant=Disabled  NCopyVariant=Disabled_SignalSpec  FilterICVariant=Disabled  IntegratorICVariant=InternalICs  ExternalResetVariant=Disabled  TRSumVariant=Passthrough  SumFdbkVariant=Disabled  SumVariant=Sum_PI  TsampFilterVariant=InternalTs  TsampNgainVariant=Passthrough  TsampIntegralVariant=Disabled_SignalSpec  ExternalSaturationOutDataTypeStr=Inherit: Same as second input  DerivativeSourceVariant=Disabled  PreIntVariant=InternalPreInt
  Sqrt : Sqrt
  Sum : Sum  Inputs=|+-
  Sum1 : Sum  Inputs=|+-
  Sum2 : Sum  Inputs=|++-
  Sum4 : Sum  Inputs=-+
  Sum5 : Sum  Inputs=+-|
  Sum8 : Sum  Inputs=++|
  dq alpha conversion : Subsystem
  Vmod : Outport
  wires:
  Sum4/1 -> PID IQ/1, Gain/1  "Iq err"
  Sum1/1 -> "PID ID "/1, Gain2/1  "Id err"
  PID IQ/1 -> Sum8/1  "Vq ref"
  Phase/1 -> dq alpha conversion/3(Phase)  "phase"
  "PID ID "/1 -> Sum2/2  "Vd ref"
  Vdc/1 -> Display/1, Sum5/2  "Vdc"
  dq alpha conversion/1(Out1) -> Vmod/1  "Vmod"
  Sum5/1 -> PID VDC/1
  Gain/1 -> Sum2/3
  Gain2/1 -> Sum8/2
  Id/1 -> Sum1/2
  Iq/1 -> Sum4/1
  Sum2/1 -> Display1/1, dq alpha conversion/1(Vd control)  "Vd control"
  Sum8/1 -> dq alpha conversion/2(Vq control), Display2/1  "Vqcontrol"
  Vd/1 -> Gain4/1, Sum2/1
  Divide/1 -> PID VQ/1
  Qmeas/1 -> Sum/2
  Sum/1 -> Divide/2
  Gain4/1 -> Divide/1
  Constant1/1 -> Divide1/1
  Divide1/1 -> Sqrt/1
  Sqrt/1 -> Sum5/1
  PID VQ/1 -> Sum4/2  "Iq ref"
  PID VDC/1 -> Sum1/1  "Id ref"
  Constant/1 -> Divide1/2
  Constant2/1 -> Sum/1

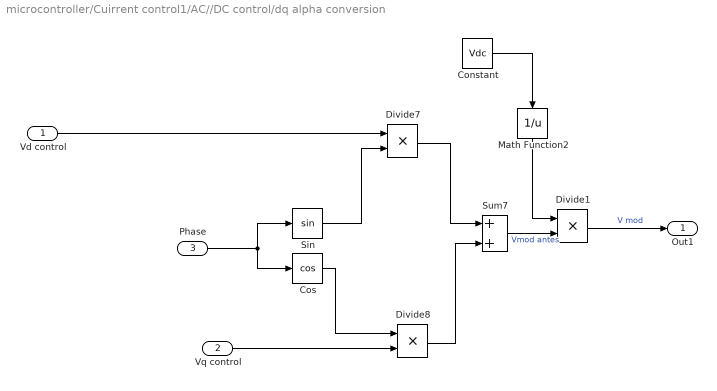
== system microcontroller/Cuirrent control1/AC//DC control/dq alpha conversion ==
  Vd control : Inport
  Vq control : Inport  Port=2
  Phase : Inport  Port=3
  Constant : Constant  Value=Vdc
  Cos : Trigonometry  Operator=cos
  Divide1 : Product  Inputs=**
  Divide7 : Product  Inputs=**
  Divide8 : Product  Inputs=**
  Math Function2 : Math  Operator=reciprocal
  Sin : Trigonometry
  Sum7 : Sum
  Out1 : Outport
  wires:
  Cos/1 -> Divide8/1
  Sin/1 -> Divide7/2
  Vd control/1 -> Divide7/1
  Divide8/1 -> Sum7/2
  Divide7/1 -> Sum7/1
  Phase/1 -> Cos/1, Sin/1
  Vq control/1 -> Divide8/2
  Sum7/1 -> Divide1/2  "Vmod antes"
  Divide1/1 -> Out1/1  "V mod"
  Math Function2/1 -> Divide1/1
  Constant/1 -> Math Function2/1
